simulink model "HyperscaleDataCenter"  (R2025b)
settings: Solver=VariableStepAuto  StartTime=0.0  StopTime=10  FixedStep=5e-5  RelTol=1e-4
PostLoadFcn:
  | HyperscaleDataCenterParam
values from neighbouring files (symbols this model uses):
  baseVoltageDC = 800    [DataCenterBBUParam.m]    (also in HyperscaleDataCenterParam.m; UPSBESSParam.m)
  bess_Ki = bess.controller.Ki    [SSTBESSParam.m]
  bess_Kp = bess.controller.Kp    [SSTBESSParam.m]
  droopGain = 0.02    [HyperscaleDataCenterParam.m]    (also in SSTBESSParam.m; UPSBESSParam.m)
  peakShavingPowerLimit = 800e3    (= 800000)    [HyperscaleDataCenterParam.m]
  powerTau = 0.005    [HyperscaleDataCenterParam.m]
  Prated_batt = 40e3    (= 40000)    [HyperscaleDataCenterParam.m]
  tauPS = 0.1    [HyperscaleDataCenterParam.m]
  Ts = 50e-6    (= 5e-05)    [BBUParam.m]    (also in DataCenterBBUParam.m; HyperscaleDataCenterParam.m)
  Ts_PS = 1e-3    (= 0.001)    [HyperscaleDataCenterParam.m]
undefined symbols (not defined in the file or in its folder): bbu, DiscIntNeverNeededParam, dspblkCoreblockFVToolHelper, ee_sli_rtmsupport, gcbh, grid, rack, sst, ups
libraries: fl_lib x80, nesl_utility x42, datacenter_lib x20, ee_lib x17, simulink x10, eeGeneralControl x9, slpidlib x6, microgridRenewables_lib x4, eeTransforms x4, batteryecm_lib x3, eeSinusoidalMeasurementV2 x2, simulink_extras x1
(part 1 of 5)
settings Model: SimulationMode=accelerator  Creator=skota  LastModifiedBy=skota
settings SolverCC: ZeroCrossAlgorithm=Adaptive
settings DataIOCC: InitialState=xBalanced
settings DebuggingCC: MinStepSizeMsg=none
settings SimscapeCC: SimscapeNominalValues="[{\"value\":\"1\",\"unit\":\"A\"},{\"value\":\"1\",\"unit\":\"bar\"},{\"value\":\"1\",\"unit\":\"cm^2\"},{\"value\":\"1\",\"unit\":\"cm^3/s\"},{\"value\":\"1\",\"unit\":\"kJ/kg\"},{\"value\":\"1\",\"unit\":\"kW\"},{\"value\":\"1\",\"unit\":\"l\"},{\"value\":\"1\",\"unit\":\"N\"},{\"value\":\"1\",\"unit\":\"N*m\"},{\"value\":\"1\",\"unit\":\"V\"},{\"value\":\"0.001\",\"unit\":\"Wb\"}]"  SimscapeLogDataHistory=10000.0

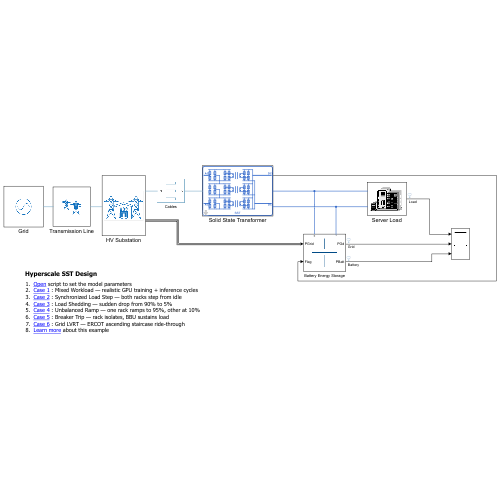
[thumbnail: Simulink's stored preview of the top-level diagram]
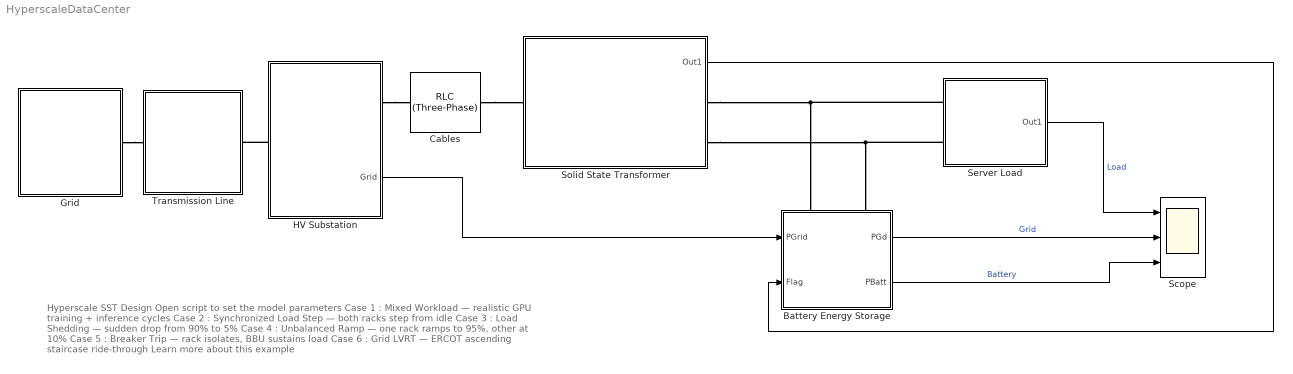
== system HyperscaleDataCenter ==
  note: Hyperscale SST Design
      | Open script to set the model parameters
      | Case 1 : Mixed Workload — realistic GPU training + inference cycles
      | Case 2 : Synchronized Load Step — both racks step from idle
      | Case 3 : Load Shedding — sudden drop from 90% to 5%
      | Case 4 : Unbalanced Ramp — one rack ramps to 95%, other at 10%
      | Case 5 : Breaker Trip — rack isolates, BBU sustains load
      | Case 6 : Grid LVRT — ERCOT ascending staircase ride-through
      | Learn more about this example
  Battery Energy Storage : Subsystem
      settings: PortSchema="{\"entries\":[{\"content\":{\"sides\":[{\"content\":{\"connectorIds\":[\"LConn1\",\"LConn2\"]},\"type\":\"ConnectorPlacement.EquallySpacedRectSide\",\"uuid\":\"f30d4562-66db-40aa-a311-a092df84fe5e\"},{\"content\":{\"side\":\"RIGHT\"},\"type\":\"ConnectorPlacement.EquallySpacedRectSide\",\"uuid\":\"82020e0e-30c9-451f-87cf-8a5183405c63\"},{\"content\":{\"connectorIds\":[\"In1\",\"In2\"],\"side\":\"TOP\"},\"type\":\"ConnectorPlacement.EquallySpacedRectSide\",\"uuid\":\"d7b483c7-3846-444d-bee9-68afc8ec1fc3\"},{\"content\":{\"connectorIds\":[\"Out1\",\"Out2\"],\"side\":\"BOTTOM\"},\"type\":\"ConnectorPlacement.EquallySpacedRectSide\",\"uuid\":\"677d4972-f2c3-4679-96cc-fb4a4809ac22\"}]},\"type\":\"ConnectorPlacement.EquallySpacedConnector\",\"uuid\":\"2e044c4a-d8de-4d2a-b140-ec8718812782\"}],\"packageUris\":[\"http://schema.mathworks.com/mf0/Connector/R2020b\"],\"version\":\"1.0\"}"
      mask Display: image('DCBusbattery_1.png');
  Cables : ee_lib/Passive/RLC Assemblies/RLC (Three-Phase)  port_option=ee.enum.threePhasePort.composite  component_structure=ee.enum.rlc.structure.SeriesRL  R=1e-3 Ohm  L=1e-5 H  C=1e-6 F  R_parasitic=0 Ohm  G_parasitic=0 1/Ohm  IL_specify=on  IL_priority=None  IL=[0, 0, 0] A  IL_nominal_specify=off  IL_nominal_value=1  IL_nominal_unit=A  VC_specify=off  VC_priority=High  VC=[0, 0, 0] V  VC_nominal_specify=off  VC_nominal_value=1  VC_nominal_unit=V
      settings: InternalSimscapePortConfiguration="{\"Bottom\":[],\"Left\":[{\"id\":\"N1\",\"label\":\"~1\",\"type\":\"foundation.electrical.three_phase\"}],\"Right\":[{\"id\":\"N2\",\"label\":\"~2\",\"type\":\"foundation.electrical.three_phase\"}],\"Top\":[]}"
  Grid : Subsystem
  HV Substation : Subsystem
      settings: PortSchema="{\"entries\":[{\"content\":{\"sides\":[{\"content\":{\"connectorIds\":[\"LConn1\"]},\"type\":\"ConnectorPlacement.EquallySpacedRectSide\",\"uuid\":\"cf02143b-cb97-440a-93ce-8a413170b7c0\"},{\"content\":{\"connectorIds\":[\"RConn1\",\"Out1\"],\"side\":\"RIGHT\"},\"type\":\"ConnectorPlacement.EquallySpacedRectSide\",\"uuid\":\"e82f4f93-e397-4fd2-8ad6-51f8e1dce17a\"},{\"content\":{\"side\":\"TOP\"},\"type\":\"ConnectorPlacement.EquallySpacedRectSide\",\"uuid\":\"5284a86a-a773-4d71-bb38-460e3da41d4c\"}]},\"type\":\"ConnectorPlacement.EquallySpacedConnector\",\"uuid\":\"36d9daed-9f92-41bd-b078-b520288a69b1\"}],\"packageUris\":[\"http://schema.mathworks.com/mf0/Connector/R2020b\"],\"version\":\"1.0\"}"
  Scope : Scope  NumInputPorts=3
      settings: ActiveDisplayYMinimum=-1.6618094800018679  ActiveDisplayYMaximum=14.956285320010076  DataLoggingVariableName=ScopeData3
  Server Load : Subsystem
      mask Display: image('datacenter.png');
  Solid State Transformer : Subsystem  mask(Solid State Transformer){inputVoltage=sst.inputVoltage, dcBusVoltage=sst.chb.dcBusVoltage, dcOutputVoltage=sst.dcOutputVoltage, frequency=sst.frequency, numModules=sst.chb.numModules, Kp_dab=sst.dab.kp, Ki_dab=sst.dab.ki, dab_sat_upper=sst.dab.upperLimit, dab_sat_lower=sst.dab.lowerLimit, dcBusCapacitance=sst.chb.dcBusCapacitance, filterInductance=sst.filter.inductance, filterResistance=sst.filter.resistance, dab_sampleTime=sst.dab.sampleTime, Vdc_init=sst.chb.Vdc_init}
      mask prompts: inputVoltage "Input Voltage - Phase to Phase RMS (V)"; dcBusVoltage "DC Bus Voltage per Module (V)"; dcOutputVoltage "DC Output Voltage (V)"; frequency "Grid Frequency (Hz)"; numModules "Number of CHB Modules per Phase"; Kp_dab "Proportional Gain (Kp)"; Ki_dab "Integral Gain (Ki)"; dab_sat_upper "Phase Shift Upper Limit"; dab_sat_lower "Phase Shift Lower Limit"; dcBusCapacitance "DC Bus Capacitance (F)"; filterInductance "Filter Inductance (H)"; filterResistance "Filter Resistance (Ohm)"; dab_sampleTime "DAB sample time (s)"; Vdc_init "Initial DC bus voltage (V)"
      mask help: Solid State Transformer with CHB rectifier and DAB DC-DC converters. Three-phase input, isolated DC output.
      mask init:
      | % SST Mask Initialization
      | % Propagate DAB PI gains to all 9 DAB controllers
      | phases = {'Subsystem1', 'Subsystem2', 'Subsystem3'};
      | 
      | % Support per-phase capacitance: scalar or [Ca Cb Cc] vector
      | if isscalar(dcBusCapacitance)
      |     capPerPhase = dcBusCapacitance * [1 1 1];
      | else
      |     capPerPhase = dcBusCapacitance;
      | end
      | 
      | % Support per-phase initial voltage: scalar or [Va Vb Vc] vector
      | if isscalar(Vdc_init)
      |     vInitPerPhase = Vdc_init * [1 1 1];
      | else
      |     vInitPerPhase = Vdc_init;
      | end
      | 
      | for p = 1:3
      |     % Propagate DC bus capacitance (per-phase)
      |     caps = {'Capacitor', 'Capacitor1', 'Capacitor2'};
      |     for c = 1:3
      |         capPath = [gcb, '/Converters/', phases{p}, '/', caps{c}];
      |         set_param(capPath, 'c', num2str(capPerPhase(p)));
      |         set_param(capPath, 'vc', num2str(vInitPerPhase(p)));
      |     end
      | end
      | 
      | % Propagate filter parameters
      | rlPath = [gcb, '/Filter & AC measurements/RL filter'];
      | set_param(rlPath, 'L', num2str(filterInductance));
      | set_param(rlPath, 'R', num2str(filterResistance));
      settings: CopyFcn=set_param(gcbh,'LinkStatus','none');
      mask Help: web("DocumentationSolidStateTransformer.html")
      mask DialogControl GeneralTab Prompt: General
      mask DialogControl PFCControlTab Prompt: PFC Control
      mask DialogControl openPFCController Prompt: Edit PFC Controller
      mask DialogControl openPFCController Callback:
      | blockPath = [gcb,'/PFC Rectifier Controller'];
      | open_system(blockPath, 'mask');
      mask DialogControl HBridgeTab Prompt: H-Bridge
      mask DialogControl openCHBBlock Prompt: Edit CHB Phase Leg Parameters
      mask DialogControl openCHBBlock Callback:
      | blockPath = [gcb,'/Converters/Subsystem1/CHB Phase Leg' char(10) '(Average Model)'];
      | open_system(blockPath, 'mask');
      mask DialogControl DABTab Prompt: DAB
      mask DialogControl openDABBlock Prompt: Edit DAB Parameters
      mask DialogControl openDABBlock Callback:
      | blockPath = [gcb,'/Converters/Subsystem1/DAB Generalized' char(10) 'Average Model'];
      | open_system(blockPath, 'mask');
      mask Display: image('sst_icon.svg')
  Transmission Line : Subsystem
  wires:
  Solid State Transformer/1(Out1) -> Battery Energy Storage/2(Flag)
  HV Substation/1(Grid) -> Battery Energy Storage/1(PGrid)
  Battery Energy Storage/1(PGd) -> Scope/2  "Grid"
  Server Load/1(Out1) -> Scope/1  "Load"
  Battery Energy Storage/2(PBatt) -> Scope/3  "Battery"
  connections:
  Server Load/LConn1 -- Solid State Transformer/RConn1 -- Battery Energy Storage/LConn1
  Server Load/LConn2 -- Solid State Transformer/RConn2 -- Battery Energy Storage/LConn2
  HV Substation/RConn1 -- Cables/LConn1
  HV Substation/LConn1 -- Transmission Line/LConn1
  Cables/RConn1 -- Solid State Transformer/LConn1
  Grid/LConn1 -- Transmission Line/RConn1

== system HyperscaleDataCenter/Battery Energy Storage ==
  PGrid : Inport
  Flag : Inport  Port=2
  BESS : Subsystem
      settings: PortSchema="{\"entries\":[{\"content\":{\"sides\":[{\"content\":{\"connectorIds\":[\"LConn1\",\"In1\",\"In2\",\"In3\",\"In4\"]},\"type\":\"ConnectorPlacement.EquallySpacedRectSide\",\"uuid\":\"9f38bdfa-ed37-47de-aef9-0aa02e5d3e08\"},{\"content\":{\"connectorIds\":[\"RConn1\",\"Out1\",\"Out2\",\"Out3\",\"Out4\"],\"side\":\"RIGHT\"},\"type\":\"ConnectorPlacement.EquallySpacedRectSide\",\"uuid\":\"6d834933-82aa-469c-9fa6-18422aee79dd\"},{\"content\":{\"side\":\"TOP\"},\"type\":\"ConnectorPlacement.EquallySpacedRectSide\",\"uuid\":\"a95e7d3c-3686-4ca2-bd1f-73a692834c20\"}]},\"type\":\"ConnectorPlacement.EquallySpacedConnector\",\"uuid\":\"a3e1c48b-7b54-4503-b239-4407a5dae286\"}],\"packageUris\":[\"http://schema.mathworks.com/mf0/Connector/R2020b\"],\"version\":\"1.0\"}"
  Bus Selector : BusSelector  OutputSignals=P,voltage
  DC Bus Voltage Sensor : fl_lib/Electrical/Electrical Sensors/Voltage Sensor
  PS-Simulink Converter : nesl_utility/PS-Simulink Converter  PhysicalDomain=network_engine_domain  SubClassName=ps_output  LeftPortType=input  RightPortType=output  PseudoPeriodic=off  Frequencies=[]  VectorFormat=inherit  Unit=inherit  AffineConversion=off
  Peak Shaving Controller : Subsystem
  Terminator : Terminator
  Terminator1 : Terminator
  Terminator2 : Terminator
  Vdc Delay : UnitDelay  InitialCondition=800  SampleTime=-1
  + : PMIOPort  Side=Left
  - : PMIOPort  Port=2  Side=Left
  PGd : Outport
  PBatt : Outport  Port=2
  wires:
  BESS/3(IDCDC) -> Terminator2/1
  BESS/1(Ibatt) -> Terminator/1
  BESS/2(SOC) -> Terminator1/1
  Vdc Delay/1 -> BESS/1(Vdc)
  PS-Simulink Converter/1 -> Vdc Delay/1
  Peak Shaving Controller/1(iRef_pu) -> BESS/2(iPeakShave)
  PGrid/1 -> Bus Selector/1
  Bus Selector/1 -> PGd/1, Peak Shaving Controller/1(Pgrid)  "<P>"
  BESS/4(PBatt) -> PBatt/1
  Bus Selector/2 -> BESS/3(Vac)  "<voltage>"
  Flag/1 -> BESS/4(Flag)
  connections:
  BESS/LConn1 -- DC Bus Voltage Sensor/LConn1 -- +/RConn1
  DC Bus Voltage Sensor/RConn2 -- -/RConn1 -- BESS/RConn1
  PS-Simulink Converter/LConn1 -- DC Bus Voltage Sensor/RConn1

== system HyperscaleDataCenter/Grid ==
  Controlled Voltage Source (Three-Phase) : ee_lib/Sources/Controlled Voltage Source (Three-Phase)  input_option=ee.enum.inputType.singleFreqAC  FRated=60 Hz
      settings: InternalSimscapePortConfiguration="{\"Bottom\":[],\"Left\":[{\"id\":\"Vt\",\"label\":\"Vt\",\"type\":\"input\"},{\"id\":\"ph\",\"label\":\"ph\",\"type\":\"input\"},{\"id\":\"n\",\"label\":\"n\",\"type\":\"foundation.electrical.electrical\"}],\"Right\":[{\"id\":\"N\",\"label\":\"~\",\"type\":\"foundation.electrical.three_phase\"}],\"Top\":[]}"
  Electrical Reference : fl_lib/Electrical/Electrical Elements/Electrical Reference
  Gain : Gain  Gain=grid.voltage
  LVRT Profile : FromWorkspace  VariableName=lvrtProfile  SampleTime=Ts  OutputAfterFinalValue=Holding final value
  PS Constant1 : fl_lib/Physical Signals/Sources/PS Constant  constant=0
  Simulink-PS Converter : nesl_utility/Simulink-PS Converter  PhysicalDomain=network_engine_domain  SubClassName=ps_input  LeftPortType=input  RightPortType=output  PseudoPeriodic=off  Frequencies=[]  NoiseDistribution=none  NoiseParameters=[]  Unit=1  AffineConversion=off  FilteringAndDerivatives=provide  SimscapeFilterOrder=1  InputFilterTimeConstant=0.001  UdotUserProvided=0
  Solver Configuration : nesl_utility/Solver Configuration  PhysicalDomain=network_engine_domain  SubClassName=solver  LeftPortType=input  RightPortType=generic  Tones=[]  Harmonics=[]  SimulateNoise=off  Profile=off  UseLocalSampling=off  EnableSwitchedLinearOptims=on  FrequencyDomain=off  UseCCode=off  RelTol=0.001  AbsTol=0.001  MinStep=1e-09  ToWorkspace=off  RevertToSquareIcSolve=off  NumHomotopyIterations=100  PhasorMode=off  PhasorModeNumHarmonics=1  ConsistencySolver=NEWTON_XTOL_AFTER_FTOL  IndexReductionMethod=None  DoDC=off  ResidualTolerance=1e-9  ConsistencyTolSource=GLOBAL  ConsistencyAbsTol=0.001  ConsistencyRelTol=0.001  ConsistencyTolFactor=1e-3  UseLocalSolver=on  LocalSolverChoice=NE_BACKWARD_EULER_ADVANCER  ResolveIndetEquations=off  FunctionEvalNumThread=1  LocalSolverSampleTime=5e-05  DoFixedCost=on  MaxNonlinIter=3  MaxModeIter=2  ComputeImpulses=off  ImpulseIterations=2  LinearAlgebra=auto  LinearAlgebraNumThread=0  EquationFormulation=NE_TIME_EF  DelaysMemoryBudget=1024  AutomaticFiltering=off  FilteringTimeConstant=0.001  PartitionStorageMethod=AS_NEEDED  PartitionMemoryBudget=1024  PartitionMethod=ROBUST  MultibodyUseLocalSolver=off  MultibodyLocalSolverChoice=ODE1  MultibodyLocalSolverSampleTime=0.001
  " " : PMIOPort  Side=Left
  wires:
  LVRT Profile/1 -> Gain/1
  Gain/1 -> Simulink-PS Converter/1
  connections:
  Controlled Voltage Source (Three-Phase)/LConn3 -- Electrical Reference/LConn1
  Controlled Voltage Source (Three-Phase)/RConn1 -- " "/RConn1 -- Solver Configuration/RConn1
  PS Constant1/RConn1 -- Controlled Voltage Source (Three-Phase)/LConn2
  Controlled Voltage Source (Three-Phase)/LConn1 -- Simulink-PS Converter/RConn1

== system HyperscaleDataCenter/HV Substation ==
  Circuit Breaker : Subsystem
  Delay : Delay  DelayLength=1  InitialCondition=1
  Demux : Demux  Outputs=3
  Gain : Gain  Gain=1/(sqrt(2)*grid.voltage)
  Gain1 : Gain  Gain=1/(grid.voltage)
  Line Voltage Sensor (Three-Phase)1 : ee_lib/Sensors & Transducers/Line Voltage Sensor (Three-Phase)
  PS RMS Estimator : fl_lib/Physical Signals/Periodic Operators/PS RMS Estimator  f0=60 Hz
      settings: InternalSimscapePortConfiguration="{\"Bottom\":[],\"Left\":[{\"id\":\"I\",\"label\":\"\",\"type\":\"input\"}],\"Right\":[{\"id\":\"O\",\"label\":\"\",\"type\":\"output\"}],\"Top\":[]}"
  PS-Simulink Converter : nesl_utility/PS-Simulink Converter  PhysicalDomain=network_engine_domain  SubClassName=ps_output  LeftPortType=input  RightPortType=output  PseudoPeriodic=off  Frequencies=[]  VectorFormat=inherit  Unit=inherit  AffineConversion=off
  PS-Simulink Converter1 : nesl_utility/PS-Simulink Converter  PhysicalDomain=network_engine_domain  SubClassName=ps_output  LeftPortType=input  RightPortType=output  PseudoPeriodic=off  Frequencies=[]  VectorFormat=inherit  Unit=inherit  AffineConversion=off
  Power Measurement : Subsystem
      settings: PortSchema="{\"entries\":[{\"content\":{\"sides\":[{\"content\":{\"connectorIds\":[\"LConn1\"]},\"type\":\"ConnectorPlacement.EquallySpacedRectSide\",\"uuid\":\"0c8863a2-a78f-4a73-a820-c6aa5bdc2133\"},{\"content\":{\"connectorIds\":[\"RConn1\"],\"side\":\"RIGHT\"},\"type\":\"ConnectorPlacement.EquallySpacedRectSide\",\"uuid\":\"2028a368-e468-46fb-8c3f-9ce74e7f0a45\"},{\"content\":{\"side\":\"TOP\"},\"type\":\"ConnectorPlacement.EquallySpacedRectSide\",\"uuid\":\"1b144116-ac84-43c3-ac53-ab33c5b71658\"},{\"content\":{\"connectorIds\":[\"Out1\",\"Out2\"],\"side\":\"BOTTOM\"},\"type\":\"ConnectorPlacement.EquallySpacedRectSide\",\"uuid\":\"3e4d0e65-8f44-4e57-8d60-68941db834c2\"}]},\"type\":\"ConnectorPlacement.EquallySpacedConnector\",\"uuid\":\"a27c8f54-ed82-4619-aed8-d6cf5e2c28e1\"}],\"packageUris\":[\"http://schema.mathworks.com/mf0/Connector/R2020b\"],\"version\":\"1.0\"}"
      mask Display: image('measurements.png');
  Step : Step  Time=100  SampleTime=0
  Terminator : Terminator
  Transformer : Subsystem  Variant=on  VariantControlMode=label  LabelModeActiveChoice=Detailed  mask{fidelity=Detailed}
      mask prompts: fidelity "Modeling Option"
      mask TypeOptions fidelity: Detailed | Simplified
      mask Callback fidelity:
      | choice = get_param(gcb,'fidelity');
      | switch choice
      |     case 'Detailed'
      |         set_param(gcb, 'LabelModeActiveChoice', 'Detailed');
      |     case 'Simplified'
      |          set_param(gcb, 'LabelModeActiveChoice', 'Simplified');
      |     otherwise
      |         disp('Choose proper variant');
      | end
  Conn1 : PMIOPort  Side=Left
  ~ : PMIOPort  Port=2  Side=Right
  Bus Element Out : Outport  PortName=Grid  Element=P
  BusElementOut : Outport  PortName=Grid  Element=Q
  BusElementOut1 : Outport  PortName=Grid  Element=voltage
  wires:
  Power Measurement/1(Q) -> BusElementOut/1  "qGrid"
  Power Measurement/2(P) -> Bus Element Out/1  "pGrid"
  Step/1 -> Circuit Breaker/1(BRK)
  PS-Simulink Converter/1 -> Gain/1
  Gain/1 -> Terminator/1
  PS-Simulink Converter1/1 -> Gain1/1
  Gain1/1 -> Demux/1
  Demux/1 -> Delay/1
  Delay/1 -> BusElementOut1/1
  connections:
  Power Measurement/RConn1 -- Line Voltage Sensor (Three-Phase)1/LConn1 -- Transformer/LConn1
  Power Measurement/LConn1 -- Conn1/RConn1
  Circuit Breaker/LConn1 -- Transformer/RConn1
  ~/RConn1 -- Circuit Breaker/RConn1
  Line Voltage Sensor (Three-Phase)1/RConn1 -- PS RMS Estimator/LConn1 -- PS-Simulink Converter/LConn1
  PS-Simulink Converter1/LConn1 -- PS RMS Estimator/RConn1

== system HyperscaleDataCenter/Server Load ==
  Current Sensor : fl_lib/Electrical/Electrical Sensors/Current Sensor
  Gain : Gain  Gain=1/1e6
  PS-Simulink Converter : nesl_utility/PS-Simulink Converter  PhysicalDomain=network_engine_domain  SubClassName=ps_output  LeftPortType=input  RightPortType=output  PseudoPeriodic=off  Frequencies=[]  VectorFormat=inherit  Unit=inherit  AffineConversion=off
  PS-Simulink Converter1 : nesl_utility/PS-Simulink Converter  PhysicalDomain=network_engine_domain  SubClassName=ps_output  LeftPortType=input  RightPortType=output  PseudoPeriodic=off  Frequencies=[]  VectorFormat=inherit  Unit=inherit  AffineConversion=off
  Product : Product
  Racks : Subsystem
  Voltage Sensor : fl_lib/Electrical/Electrical Sensors/Voltage Sensor
  Connection Port : PMIOPort  Side=Left
  Connection Port1 : PMIOPort  Port=2  Side=Left
  Out1 : Outport
  wires:
  PS-Simulink Converter/1 -> Product/2  "Vdc_800V"
  Product/1 -> Gain/1
  PS-Simulink Converter1/1 -> Product/1  "I_dc_total"
  Gain/1 -> Out1/1
  connections:
  Voltage Sensor/RConn2 -- Racks/LConn2 -- Connection Port1/RConn1
  Connection Port/RConn1 -- Current Sensor/LConn1 -- Voltage Sensor/LConn1
  PS-Simulink Converter/LConn1 -- Voltage Sensor/RConn1
  PS-Simulink Converter1/LConn1 -- Current Sensor/RConn1
  Racks/LConn1 -- Current Sensor/RConn2

== system HyperscaleDataCenter/Solid State Transformer ==
  note: Cascaded H-Bridge modules with DAB
  note: DAB Control
  note: Rectifier Control
  Constant1 : Constant  Value=dcBusVoltage
  Constant2 : Constant  Value=0
  Converters : Subsystem
      settings: PortSchema="{\"entries\":[{\"content\":{\"sides\":[{\"content\":{\"connectorIds\":[\"In1\",\"In2\",\"LConn1\"]},\"type\":\"ConnectorPlacement.EquallySpacedRectSide\",\"uuid\":\"3c50ecae-d327-4517-ac35-d4ccad8214d6\"},{\"content\":{\"connectorIds\":[\"RConn1\",\"RConn2\",\"Out1\",\"Out2\"],\"side\":\"RIGHT\"},\"type\":\"ConnectorPlacement.EquallySpacedRectSide\",\"uuid\":\"ce483151-8cc4-4e89-a036-44eb982feae5\"},{\"content\":{\"side\":\"TOP\"},\"type\":\"ConnectorPlacement.EquallySpacedRectSide\",\"uuid\":\"39146706-ffb9-4bd3-97cb-72551c78d2ac\"}]},\"type\":\"ConnectorPlacement.EquallySpacedConnector\",\"uuid\":\"8cf16702-94fc-4b9b-91c9-b502d0239b3b\"}],\"packageUris\":[\"http://schema.mathworks.com/mf0/Connector/R2020b\"],\"version\":\"1.0\"}"
  DAB Controller : Subsystem
  DC Voltage Balancing : Subsystem
  Filter & AC measurements : Subsystem
  PFC Rectifier Controller : Subsystem  LoadFcn=%ee_sli_rtmsupport( 'loadfcn', gcbh );  mask(PFC Rectifier Controller (Three-Phase)){Freq=sst.pfc.frequency, L=sst.pfc.filterInductance, BaseImpedance=sst.pfc.baseImpedance, KpPLL=sst.pfc.kpPLL, KiPLL=sst.pfc.kiPLL, Ts=sst.pfc.sampleTime, KpVoltage=sst.pfc.kpVoltage, KiVoltage=sst.pfc.kiVoltage, KdVoltage=sst.pfc.kdVoltage, NdVoltage=sst.pfc.NdVoltage, BaseVdc=sst.pfc.baseVdc, VoltControlUpperLimit=sst.pfc.voltageUpperLimit, VoltControlLowerLimit=sst.pfc.voltageLowerLimit, KpdCurrent=sst.pfc.kpId, KidCurrent=sst.pfc.kiId, KddCurrent=sst.pfc.kdId, IdControlUpperLimit=sst.pfc.IdUpperLimit, IdControlLowerLimit=sst.pfc.IdLowerLimit, KpqCurrent=sst.pfc.kpIq, KiqCurrent=sst.pfc.kiIq, KdqCurrent=sst.pfc.kdIq, NdCurrent=sst.pfc.NdCurrent, IqControlUpperLimit=sst.pfc.IqUpperLimit, IqControlLowerLimit=sst.pfc.IqLowerLimit}
      mask prompts: Freq "physmod:ee:library:comments:control:eeConverterControllers:SystemFrequencyHz_MP"; L "physmod:ee:library:comments:control:eeConverterControllers:ACFilterInductanceH_MP"; BaseImpedance "physmod:ee:library:comments:control:eeConverterControllers:ACSideBaseImpedanceOhm_MP"; KpPLL "physmod:ee:library:comments:control:eeConverterControllers:PLLProportionalGain_MP"; KiPLL "physmod:ee:library:comments:control:eeConverterControllers:PLLIntegralGain_MP"; Ts "physmod:ee:library:comments:control:eeConverterControllers:SampleTime1ForInherited_MP"; KpVoltage "physmod:ee:library:comments:control:eeConverterControllers:ProportionalGain_MP"; KiVoltage "physmod:ee:library:comments:control:eeConverterControllers:IntegralGain_MP"; KdVoltage "physmod:ee:library:comments:control:eeConverterControllers:DerivativeGain_MP"; NdVoltage "physmod:ee:library:comments:control:eeConverterControllers:DerivativeControllerFilterCoefficientN_MP"; BaseVdc "physmod:ee:library:comments:control:eeConverterControllers:DCBusBaseVoltageV_MP"; VoltControlUpperLimit "physmod:ee:library:comments:control:eeConverterControllers:ControllerOutputUpperLimitpu_MP"; VoltControlLowerLimit "physmod:ee:library:comments:control:eeConverterControllers:ControllerOutputLowerLimitpu_MP"; KpdCurrent "physmod:ee:library:comments:control:eeConverterControllers:IdProportionalGain_MP"; KidCurrent "physmod:ee:library:comments:control:eeConverterControllers:IdIntegralGain_MP"; KddCurrent "physmod:ee:library:comments:control:eeConverterControllers:IdDerivativeGain_MP"; IdControlUpperLimit "physmod:ee:library:comments:control:eeConverterControllers:IdControllerOutputUpperLimitpu_MP"; IdControlLowerLimit "physmod:ee:library:comments:control:eeConverterControllers:IdControllerOutputLowerLimitpu_MP"; KpqCurrent "physmod:ee:library:comments:control:eeConverterControllers:IqProportionalGain_MP"; KiqCurrent "physmod:ee:library:comments:control:eeConverterControllers:IqIntegralGain_MP"; KdqCurrent "physmod:ee:library:comments:control:eeConverterControllers:IqDerivativeGain_MP"; NdCurrent "physmod:ee:library:comments:control:eeConverterControllers:DerivativeCurrentControllerFilterCoefficientN_MP"; IqControlUpperLimit "physmod:ee:library:comments:control:eeConverterControllers:IqControllerOutputUpperLimitpu_MP"; IqControlLowerLimit "physmod:ee:library:comments:control:eeConverterControllers:IqControllerOutputLowerLimitpu_MP"
      mask help: physmod:ee:library:comments:control:eeConverterControllers:PFCRectifierController_MD
      mask init:
      | ee.mask.initializePFCController(gcb,Ts, Freq, L,BaseImpedance,KpPLL,KiPLL,KpVoltage,KiVoltage,KdVoltage,BaseVdc, NdVoltage,VoltControlUpperLimit,VoltControlLowerLimit,KpdCurrent, KidCurrent, KddCurrent, NdCurrent, IdControlUpperLimit, IdControlLowerLimit, KpqCurrent, KiqCurrent, KdqCurrent, IqControlUpperLimit, IqControlLowerLimit);
      settings: CopyFcn=%ee_sli_rtmsupport( 'copyfcn', gcbh );  DeleteFcn=ee_sli_rtmsupport( 'deletefcn', gcbh );  ModelCloseFcn=ee_sli_rtmsupport( 'modelclosefcn', gcbh );  PostSaveFcn=ee_sli_rtmsupport( 'postsavefcn', gcbh );  PreCopyFcn=ee_sli_rtmsupport( 'precopyfcn', gcbh );  OpenFcn=ee_sli_rtmsupport( 'openfcn', gcbh );  CloseFcn=%ee_sli_rtmsupport( 'closefcn', gcbh );  PreDeleteFcn=ee_sli_rtmsupport( 'predeletefcn', gcbh );
      mask Help: web(nesl_help(gcbh))
      mask DialogControl GeneralTabVal Prompt: physmod:ee:library:comments:control:eeConverterControllers:tab_General
      mask DialogControl Freq Prompt: System frequency (Hz)
      mask DialogControl L Prompt: AC filter inductance (H)
      mask DialogControl BaseImpedance Prompt: AC side base impedance (Ohm)
      mask DialogControl KpPLL Prompt: PLL proportional gain
      mask DialogControl KiPLL Prompt: PLL integral gain
      mask DialogControl Ts Prompt: Sample time (-1 for inherited)
      mask DialogControl VoltageControl Prompt: physmod:ee:library:comments:control:eeConverterControllers:tab_VoltageController
      mask DialogControl KpVoltage Prompt: Proportional gain
      mask DialogControl KiVoltage Prompt: Integral gain
      mask DialogControl KdVoltage Prompt: Derivative gain
      mask DialogControl NdVoltage Prompt: Derivative controller filter coefficient (N)
      mask DialogControl BaseVdc Prompt: DC bus base voltage (V)
      mask DialogControl VoltControlUpperLimit Prompt: Controller output upper limit (pu)
      mask DialogControl VoltControlLowerLimit Prompt: Controller output lower limit (pu)
      mask DialogControl CurrentControl Prompt: physmod:ee:library:comments:control:eeConverterControllers:tab_CurrentController
      mask DialogControl KpdCurrent Prompt: Id proportional gain
      mask DialogControl KidCurrent Prompt: Id integral gain
      mask DialogControl KddCurrent Prompt: Id derivative gain
      mask DialogControl IdControlUpperLimit Prompt: Id controller output upper limit (pu)
      mask DialogControl IdControlLowerLimit Prompt: Id controller output lower limit (pu)
      mask DialogControl KpqCurrent Prompt: Iq proportional gain
      mask DialogControl KiqCurrent Prompt: Iq integral gain
      mask DialogControl KdqCurrent Prompt: Iq derivative gain
      mask DialogControl NdCurrent Prompt: Derivative current controller filter coefficient (N)
      mask DialogControl IqControlUpperLimit Prompt: Iq controller output upper limit (pu)
      mask DialogControl IqControlLowerLimit Prompt: Iq controller output lower limit (pu)
  + : PMIOPort  Side=Right
  - : PMIOPort  Port=2  Side=Right
  ABC : PMIOPort  Port=3  Side=Left
  Out1 : Outport
  wires:
  Constant2/1 -> PFC Rectifier Controller/2(QRef (pu))
  Constant1/1 -> PFC Rectifier Controller/1(VdcRef (V))
  Filter & AC measurements/1(Vabc) -> PFC Rectifier Controller/4(VabcSens (pu))
  Converters/2(VdcMeas) -> PFC Rectifier Controller/3(VdcSens (V))
  Filter & AC measurements/2(Iabc) -> PFC Rectifier Controller/5(IabcSens (pu))
  DC Voltage Balancing/1(mabc) -> Converters/1(mabc)
  Converters/1(Vdc) -> DAB Controller/1(Vdc), DC Voltage Balancing/1(Vdc)
  DAB Controller/1(phi) -> Converters/2(phi)
  PFC Rectifier Controller/1(VabcRef (pu)) -> DC Voltage Balancing/2(VabcRef)
  PFC Rectifier Controller/2(Visualization) -> DAB Controller/2(Vac)
  PFC Rectifier Controller/3(Flag) -> Out1/1
  connections:
  Filter & AC measurements/LConn1 -- ABC/RConn1
  -/RConn1 -- Converters/RConn2
  +/RConn1 -- Converters/RConn1
  Filter & AC measurements/RConn1 -- Converters/LConn1

== system HyperscaleDataCenter/Transmission Line ==
  RLC (Three-Phase) : ee_lib/Passive/RLC Assemblies/RLC (Three-Phase)  port_option=ee.enum.threePhasePort.composite  component_structure=ee.enum.rlc.structure.SeriesRL  R=1e-2*10 Ohm  L=1e-6*10 H  C=1e-6 F  R_parasitic=0 Ohm  G_parasitic=0 1/Ohm  IL_specify=off  IL_priority=None  IL=[0, 0, 0] A  IL_nominal_specify=off  IL_nominal_value=1  IL_nominal_unit=A  VC_specify=off  VC_priority=High  VC=[0, 0, 0] V  VC_nominal_specify=off  VC_nominal_value=1  VC_nominal_unit=V
      settings: InternalSimscapePortConfiguration="{\"Bottom\":[],\"Left\":[{\"id\":\"N1\",\"label\":\"~1\",\"type\":\"foundation.electrical.three_phase\"}],\"Right\":[{\"id\":\"N2\",\"label\":\"~2\",\"type\":\"foundation.electrical.three_phase\"}],\"Top\":[]}"
  Out : PMIOPort  Side=Left
  In : PMIOPort  Port=2  Side=Right
  connections:
  RLC (Three-Phase)/LConn1 -- In/RConn1
  RLC (Three-Phase)/RConn1 -- Out/RConn1

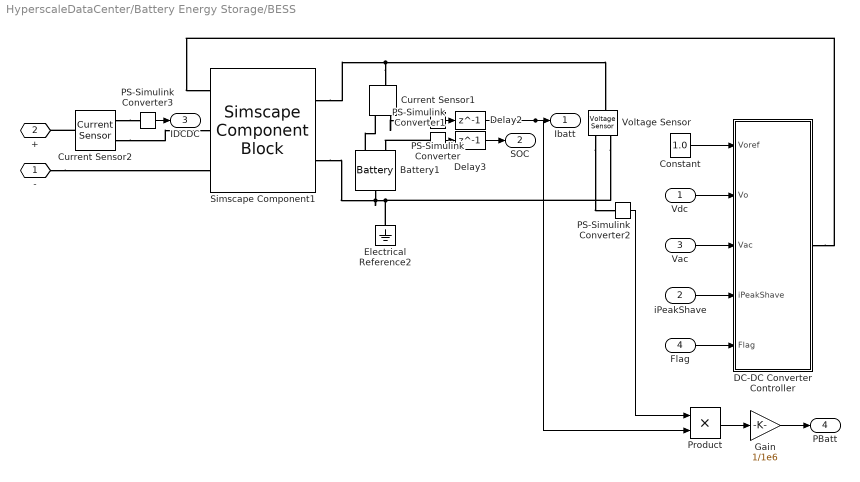
== system HyperscaleDataCenter/Battery Energy Storage/BESS ==
  Vdc : Inport
  iPeakShave : Inport  Port=2
  Vac : Inport  Port=3
  Flag : Inport  Port=4
  Battery1 : batteryecm_lib/Battery  Vnom=400 V  prm_dir=simscape.enum.battery.prm_dir.disabled  R1_dis=2 Ohm  R1_ch=2 Ohm  R1=1e-3 Ohm  prm_AH=simscape.enum.battery.prm_AH.infinite  AH=50 A*hr  V1=11.5 V  AH1=25 A*hr  prm_R2=simscape.enum.battery.prm_R2.disabled  R2=2000 Ohm  Tmeas=298.15 K  charge_measurement_port=simscape.enum.battery.enable.yes  prm_dyn=simscape.enum.battery.prm_dyn.off  Rp1=0.005 Ohm  tau1=30 s  Rp2=0.005 Ohm  tau2=30 s  Rp3=0.005 Ohm  tau3=30 s  Rp4=0.005 Ohm  tau4=30 s  Rp5=0.005 Ohm  tau5=30 s  prm_fade=simscape.enum.battery.prm_fade.disabled  N_fade=100  AH_fade=45 A*hr  R1_fade=2.02 Ohm  R1_ch_fade=2.02 Ohm  V1_fade=10.35 V  prm_age=simscape.enum.battery.prm_age.disabled  prm_age_OCV=simscape.enum.battery.prm_age_OCV.OCV  OCV_age=0.9  SOC_age=60  Tmeas_age=298.15 K  delta_time_age_vec=[0] d  temperature_age_vec=[273] K  OCV_scaling_age=2.2134e6  OCV_offset_age=1.632e6  temp_exp_age=0.515833569 V  t_exp_age=0.75  Vnom_T2=12 V  R1_T2=2.2 Ohm  R1_T2_dis=2.2 Ohm  R1_T2_ch=2.2 Ohm  V1_T2=11.4 V  R2_T2=2200 Ohm  Rp1_T2=0.005 Ohm  tau1_T2=30 s  Rp2_T2=0.005 Ohm  tau2_T2=30 s  Rp3_T2=0.005 Ohm  tau3_T2=30 s  Rp4_T2=0.005 Ohm  tau4_T2=30 s  Rp5_T2=0.005 Ohm  tau5_T2=30 s  Tmeas2=273.15 K  thermal_port=simscape.enum.thermaleffects.omit  thermal_mass=30000 J/K  i_specify=off  i_priority=None  i=0 A  i_nominal_specify=off  i_nominal_value=1  i_nominal_unit=A  v_specify=on  v_priority=None  v=400 V  v_nominal_specify=off  v_nominal_value=1  v_nominal_unit=V  charge_specify=off  charge_priority=High  charge=50 A*hr  charge_nominal_specify=off  charge_nominal_value=1  charge_nominal_unit=A*hr  num_cycles_specify=off  num_cycles_priority=High  num_cycles=0  num_cycles_nominal_specify=off  num_cycles_nominal_value=1  num_cycles_nominal_unit=1  temperature_specify=off  temperature_priority=High  temperature=298.15 K  temperature_nominal_specify=off  temperature_nominal_value=1  temperature_nominal_unit=K
      settings: InternalSimscapePortConfiguration="{\"Bottom\":[],\"Left\":[{\"id\":\"p\",\"label\":\"+\",\"type\":\"foundation.electrical.electrical\"},{\"id\":\"q\",\"label\":\"q\",\"type\":\"output\"}],\"Right\":[{\"id\":\"n\",\"label\":\"-\",\"type\":\"foundation.electrical.electrical\"}],\"Top\":[]}"
  Constant : Constant  Value=1.0
  Current Sensor1 : fl_lib/Electrical/Electrical Sensors/Current Sensor
  Current Sensor2 : fl_lib/Electrical/Electrical Sensors/Current Sensor
  DC-DC Converter Controller : Subsystem
  Delay2 : Delay  DelayLength=1  InitialCondition=400
  Delay3 : Delay  DelayLength=1  InitialCondition=400
  Electrical Reference2 : fl_lib/Electrical/Electrical Elements/Electrical Reference
  Gain : Gain  Gain=1/1e6
  PS-Simulink Converter{,1..3} (4 alike) : nesl_utility/PS-Simulink Converter  PhysicalDomain=network_engine_domain  SubClassName=ps_output  LeftPortType=input  RightPortType=output  PseudoPeriodic=off  Frequencies=[]  VectorFormat=inherit  Unit=inherit  AffineConversion=off
  Product : Product
  Simscape Component1 : SimscapeComponentBlock  SourceFile=microgridRenewables.biDirectionalConverter  ComponentPath=microgridRenewables.biDirectionalConverter  ComponentVariants="[\"microgridRenewables.biDirectionalConverter\"]"  ComponentVariantNames="[\"biDirectionalConverter\"]"  ClassName=biDirectionalConverter  SchemaVersion=1  efficiency_option=ee.enum.converters.efficiency.constant  efficiency_fixed=100  i_vec=[0, 2, 5] A  efficiency_vec=[90, 95, 98]  iL_specify=off  iL_priority=High  iL=0 A  iL_nominal_specify=off  iL_nominal_value=1  iL_nominal_unit=A  vc_specify=off  vc_priority=High  vc=0 V  vc_nominal_specify=off  vc_nominal_value=1  vc_nominal_unit=V  i1_specify=off  i1_priority=None  i1=0 A  i1_nominal_specify=off  i1_nominal_value=1  i1_nominal_unit=A  i2_specify=off  i2_priority=None  i2=0 A  i2_nominal_specify=off  i2_nominal_value=1  i2_nominal_unit=A  v1_specify=off  v1_priority=None  v1=0 V  v1_nominal_specify=off  v1_nominal_value=1  v1_nominal_unit=V  v2_specify=off  v2_priority=None  v2=0 V  v2_nominal_specify=off  v2_nominal_value=1  v2_nominal_unit=V
      settings: CopyFcn=simscape.sscblock.internal.componentBlockCallback(gcbh,'COPY')  PreCopyFcn=simscape.sscblock.internal.componentBlockCallback(gcbh,'PRECOPY')  PreDeleteFcn=simscape.sscblock.internal.componentBlockCallback(gcbh,'PREDELETE')  InternalSimscapePortConfiguration="{\"Bottom\":[],\"Left\":[{\"id\":\"Iref\",\"label\":\"Iref\",\"type\":\"input\"},{\"id\":\"p1\",\"label\":\"1+\",\"type\":\"foundation.electrical.electrical\"},{\"id\":\"n1\",\"label\":\"1-\",\"type\":\"foundation.electrical.electrical\"}],\"Right\":[{\"id\":\"p2\",\"label\":\"2+\",\"type\":\"foundation.electrical.electrical\"},{\"id\":\"n2\",\"label\":\"2-\",\"type\":\"foundation.electrical.electrical\"}],\"Top\":[]}"
      mask Type: Bi-directional DC-DC Converter
  Voltage Sensor : fl_lib/Electrical/Electrical Sensors/Voltage Sensor
  - : PMIOPort  Side=Left
  + : PMIOPort  Port=2  Side=Right
  Ibatt : Outport
  SOC : Outport  Port=2
  IDCDC : Outport  Port=3
  PBatt : Outport  Port=4
  wires:
  Vdc/1 -> DC-DC Converter Controller/2(Vo)
  Constant/1 -> DC-DC Converter Controller/1(Voref)
  PS-Simulink Converter/1 -> Delay2/1
  Delay2/1 -> Ibatt/1, Product/2
  PS-Simulink Converter1/1 -> Delay3/1
  Delay3/1 -> SOC/1
  PS-Simulink Converter2/1 -> Product/1
  PS-Simulink Converter3/1 -> IDCDC/1
  iPeakShave/1 -> DC-DC Converter Controller/4(iPeakShave)
  Product/1 -> Gain/1
  Gain/1 -> PBatt/1
  Vac/1 -> DC-DC Converter Controller/3(Vac)
  Flag/1 -> DC-DC Converter Controller/5(Flag)
  connections:
  Electrical Reference2/LConn1 -- Battery1/RConn1 -- Simscape Component1/RConn2 -- Voltage Sensor/RConn2
  Battery1/LConn1 -- Current Sensor1/RConn2
  Voltage Sensor/RConn1 -- PS-Simulink Converter2/LConn1
  -/RConn1 -- Simscape Component1/LConn3
  DC-DC Converter Controller/RConn1 -- Simscape Component1/LConn1
  Current Sensor1/RConn1 -- PS-Simulink Converter/LConn1
  PS-Simulink Converter1/LConn1 -- Battery1/LConn2
  Current Sensor2/RConn2 -- Simscape Component1/LConn2
  Current Sensor2/LConn1 -- +/RConn1
  Current Sensor2/RConn1 -- PS-Simulink Converter3/LConn1
  Current Sensor1/LConn1 -- Simscape Component1/RConn1 -- Voltage Sensor/LConn1

== system HyperscaleDataCenter/Battery Energy Storage/Peak Shaving Controller ==
  Pgrid : Inport
  Gain : Gain  Gain=1e6
  LPF : DiscreteTransferFcn  LoadFcn=dspblkCoreblockFVToolHelper(gcbh,'load');  Numerator=[tauPS]  Denominator=[1 tauPS]  SampleTime=Ts_PS
      settings: CopyFcn=dspblkCoreblockFVToolHelper(gcbh,'copy');  DeleteFcn=dspblkCoreblockFVToolHelper(gcbh,'close');  ModelCloseFcn=dspblkCoreblockFVToolHelper(gcbh,'close');  PreSaveFcn=dspblkCoreblockFVToolHelper(gcbh,'presave');  PostSaveFcn=dspblkCoreblockFVToolHelper(gcbh,'postsave');  CloseFcn=dspblkCoreblockFVToolHelper(gcbh,'close');
  Normalize : Gain  Gain=-1/Prated_batt
  Power Limit : Constant  Value=peakShavingPowerLimit
  Saturation : Saturate  UpperLimit=0  LowerLimit=-1
  Sum : Sum  Inputs=+-
  iRef_pu : Outport
  wires:
  Pgrid/1 -> Gain/1
  Power Limit/1 -> Sum/2
  Sum/1 -> Normalize/1
  Normalize/1 -> LPF/1
  LPF/1 -> Saturation/1
  Saturation/1 -> iRef_pu/1
  Gain/1 -> Sum/1

== system HyperscaleDataCenter/HV Substation/Circuit Breaker ==
  BRK : Inport
  Data Type Conversion : DataTypeConversion  OutDataTypeStr=double  SaturateOnIntegerOverflow=off  RndMeth=Floor
  Open Resistance : Gain  Gain=5e6
  Phase Splitter : ee_lib/Connectors & References/Phase Splitter
  Phase Splitter1 : ee_lib/Connectors & References/Phase Splitter
  Simulink-PS Converter : nesl_utility/Simulink-PS Converter  PhysicalDomain=network_engine_domain  SubClassName=ps_input  LeftPortType=input  RightPortType=output  PseudoPeriodic=off  Frequencies=[]  NoiseDistribution=none  NoiseParameters=[]  Unit=1  AffineConversion=off  FilteringAndDerivatives=provide  SimscapeFilterOrder=1  InputFilterTimeConstant=0.001  UdotUserProvided=0
  Variable Resistor : fl_lib/Electrical/Electrical Elements/Variable Resistor  Rmin=1e-3 Ohm  thermalEnable=false  thermal_mass=1 J/K  i_specify=on  i_priority=None  i=0 A  i_nominal_specify=off  i_nominal_value=1  i_nominal_unit=A  v_specify=off  v_priority=None  v=0 V  v_nominal_specify=off  v_nominal_value=1  v_nominal_unit=V  T_specify=off  T_priority=None  T=300 K  T_nominal_specify=off  T_nominal_value=1  T_nominal_unit=K
  Variable Resistor1 : fl_lib/Electrical/Electrical Elements/Variable Resistor  Rmin=1e-3 Ohm  thermalEnable=false  thermal_mass=1 J/K  i_specify=on  i_priority=None  i=0 A  i_nominal_specify=off  i_nominal_value=1  i_nominal_unit=A  v_specify=off  v_priority=None  v=0 V  v_nominal_specify=off  v_nominal_value=1  v_nominal_unit=V  T_specify=off  T_priority=None  T=300 K  T_nominal_specify=off  T_nominal_value=1  T_nominal_unit=K
  Variable Resistor2 : fl_lib/Electrical/Electrical Elements/Variable Resistor  Rmin=1e-3 Ohm  thermalEnable=false  thermal_mass=1 J/K  i_specify=on  i_priority=None  i=0 A  i_nominal_specify=off  i_nominal_value=1  i_nominal_unit=A  v_specify=off  v_priority=None  v=0 V  v_nominal_specify=off  v_nominal_value=1  v_nominal_unit=V  T_specify=off  T_priority=None  T=300 K  T_nominal_specify=off  T_nominal_value=1  T_nominal_unit=K
  In : PMIOPort  Side=Left
  ~ : PMIOPort  Port=2  Side=Right
  wires:
  Data Type Conversion/1 -> Open Resistance/1
  BRK/1 -> Data Type Conversion/1
  Open Resistance/1 -> Simulink-PS Converter/1
  connections:
  Phase Splitter1/RConn2 -- Variable Resistor1/RConn1
  Variable Resistor1/LConn2 -- Phase Splitter/RConn2
  Phase Splitter1/RConn3 -- Variable Resistor2/RConn1
  Phase Splitter/RConn1 -- Variable Resistor/LConn2
  Variable Resistor2/LConn2 -- Phase Splitter/RConn3
  Phase Splitter1/RConn1 -- Variable Resistor/RConn1
  Phase Splitter1/LConn1 -- ~/RConn1
  Variable Resistor/LConn1 -- Simulink-PS Converter/RConn1 -- Variable Resistor2/LConn1 -- Variable Resistor1/LConn1
  Phase Splitter/LConn1 -- In/RConn1

== system HyperscaleDataCenter/HV Substation/Power Measurement ==
  Low-Pass Filter (Discrete or Continuous) : eeGeneralControl/Low-Pass Filter (Discrete or Continuous)  K=1  T=powerTau  B=inf  A=-inf  init_option=Inherited from block input  x0=0  Ts=-1
  Low-Pass Filter (Discrete or Continuous)1 : eeGeneralControl/Low-Pass Filter (Discrete or Continuous)  K=1  T=powerTau  B=inf  A=-inf  init_option=Inherited from block input  x0=0  Ts=-1
  PS-Simulink Converter2 : nesl_utility/PS-Simulink Converter  PhysicalDomain=network_engine_domain  SubClassName=ps_output  LeftPortType=input  RightPortType=output  PseudoPeriodic=off  Frequencies=[]  VectorFormat=inherit  Unit=MW  AffineConversion=off
  PS-Simulink Converter3 : nesl_utility/PS-Simulink Converter  PhysicalDomain=network_engine_domain  SubClassName=ps_output  LeftPortType=input  RightPortType=output  PseudoPeriodic=off  Frequencies=[]  VectorFormat=inherit  Unit=MW  AffineConversion=off
  Power Sensor (Three-Phase) : ee_lib/Sensors & Transducers/Power Sensor (Three-Phase)  load_type=ee.enum.passive.type_balanced.balanced  f0=60 Hz
      settings: InternalSimscapePortConfiguration="{\"Bottom\":[],\"Left\":[{\"id\":\"N1\",\"label\":\"~1\",\"type\":\"foundation.electrical.three_phase\"}],\"Right\":[{\"id\":\"N2\",\"label\":\"~2\",\"type\":\"foundation.electrical.three_phase\"}],\"Top\":[{\"id\":\"Pm\",\"label\":\"P\",\"type\":\"output\"},{\"id\":\"Qm\",\"label\":\"Q\",\"type\":\"output\"}]}"
  In : PMIOPort  Side=Left
  Out : PMIOPort  Port=2  Side=Right
  Q : Outport
  P : Outport  Port=2
  wires:
  PS-Simulink Converter2/1 -> Low-Pass Filter (Discrete or Continuous)/1
  Low-Pass Filter (Discrete or Continuous)/1 -> P/1
  PS-Simulink Converter3/1 -> Low-Pass Filter (Discrete or Continuous)1/1
  Low-Pass Filter (Discrete or Continuous)1/1 -> Q/1
  connections:
  Power Sensor (Three-Phase)/LConn1 -- In/RConn1
  Power Sensor (Three-Phase)/RConn1 -- Out/RConn1
  Power Sensor (Three-Phase)/LConn2 -- PS-Simulink Converter2/LConn1
  Power Sensor (Three-Phase)/LConn3 -- PS-Simulink Converter3/LConn1

== system HyperscaleDataCenter/HV Substation/Transformer ==
  Detailed : Subsystem  VariantControl=Detailed
  Simplified : Subsystem  VariantControl=Simplified  mask{windingRatio=13500/6600}
      mask prompts: windingRatio "Winding ratio"
      mask DialogControl Container4 Prompt: General
  In : PMIOPort  Side=Left
  Out : PMIOPort  Port=2  Side=Right
